simulink model "Framework"  (R2017b)
settings: Solver=ode1  StartTime=0.0  StopTime=Inf  FixedStep=0.001  RelTol=1e-3
PostLoadFcn:
  | , if any(exist('dsrtsu_mdlpostloadfcn', 'file') == [2, 3, 6]), try dsrtsu_mdlpostloadfcn('Execute', bdroot); catch fprintf('Error in PostLoadFcn (dsrtsu_mdlpostloadfcn) for model "%s":\n %s\n', bdroot, lasterr); end, end,
InitFcn:
  | Parameter_INIT
undefined symbols (not defined in the file or in its folder): drive, motor
libraries: rtican x46, simulink x8, neural x1
(part 10 of 10)

== system Framework/duty cycle RR/Transmit OK Detection ==
  note: This subsystem surveys if the sending of the TX message is successful and if it meets the
      | requirements concerning the regularity of the sending.
      |
      | If for 5 consecutive execution steps the message could not be successfully sent the 'TX Warn'
      | output is set to 1. Also, the message is expected to be sent every 50 ms approximatively. If this
      | condition is not met 5 times consecutively the 'TX Warn' output is set to 1.
  TX status : Inport
  TX delta time : Inport  Port=2
  Delta time limit : Constant  Value=0.055
  Delta time limit exceeded : RelationalOperator  RndMeth=Nearest  InputSameDT=on
  Mem{1..4} (4 alike) : Memory
  OR : Logic  Operator=OR
  Prev. msg. not sent : RelationalOperator  Operator=~=  RndMeth=Nearest  InputSameDT=on
  Prev. msg. sent value : Constant
  Warn : Logic  Inputs=5
  TX Warn : Outport
  wires:
  TX delta time/1 -> Delta time limit exceeded/1
  Delta time limit/1 -> Delta time limit exceeded/2
  Prev. msg. sent value/1 -> Prev. msg. not sent/2
  TX status/1 -> Prev. msg. not sent/1
  Prev. msg. not sent/1 -> OR/1
  Delta time limit exceeded/1 -> OR/2
  OR/1 -> Mem1/1, Warn/1
  Mem1/1 -> Mem2/1, Warn/2
  Mem2/1 -> Mem3/1, Warn/3
  Mem3/1 -> Mem4/1, Warn/4
  Mem4/1 -> Warn/5
  Warn/1 -> TX Warn/1

== system Framework/position FL/Transmit OK Detection ==
  note: This subsystem surveys if the sending of the TX message is successful and if it meets the
      | requirements concerning the regularity of the sending.
      |
      | If for 5 consecutive execution steps the message could not be successfully sent the 'TX Warn'
      | output is set to 1. Also, the message is expected to be sent every 50 ms approximatively. If this
      | condition is not met 5 times consecutively the 'TX Warn' output is set to 1.
  TX status : Inport
  TX delta time : Inport  Port=2
  Delta time limit : Constant  Value=0.055
  Delta time limit exceeded : RelationalOperator  RndMeth=Nearest  InputSameDT=on
  Mem{1..4} (4 alike) : Memory
  OR : Logic  Operator=OR
  Prev. msg. not sent : RelationalOperator  Operator=~=  RndMeth=Nearest  InputSameDT=on
  Prev. msg. sent value : Constant
  Warn : Logic  Inputs=5
  TX Warn : Outport
  wires:
  TX delta time/1 -> Delta time limit exceeded/1
  Delta time limit/1 -> Delta time limit exceeded/2
  Prev. msg. sent value/1 -> Prev. msg. not sent/2
  TX status/1 -> Prev. msg. not sent/1
  Prev. msg. not sent/1 -> OR/1
  Delta time limit exceeded/1 -> OR/2
  OR/1 -> Mem1/1, Warn/1
  Mem1/1 -> Mem2/1, Warn/2
  Mem2/1 -> Mem3/1, Warn/3
  Mem3/1 -> Mem4/1, Warn/4
  Mem4/1 -> Warn/5
  Warn/1 -> TX Warn/1

== system Framework/position FR/Transmit OK Detection ==
  note: This subsystem surveys if the sending of the TX message is successful and if it meets the
      | requirements concerning the regularity of the sending.
      |
      | If for 5 consecutive execution steps the message could not be successfully sent the 'TX Warn'
      | output is set to 1. Also, the message is expected to be sent every 50 ms approximatively. If this
      | condition is not met 5 times consecutively the 'TX Warn' output is set to 1.
  TX status : Inport
  TX delta time : Inport  Port=2
  Delta time limit : Constant  Value=0.055
  Delta time limit exceeded : RelationalOperator  RndMeth=Nearest  InputSameDT=on
  Mem{1..4} (4 alike) : Memory
  OR : Logic  Operator=OR
  Prev. msg. not sent : RelationalOperator  Operator=~=  RndMeth=Nearest  InputSameDT=on
  Prev. msg. sent value : Constant
  Warn : Logic  Inputs=5
  TX Warn : Outport
  wires:
  TX delta time/1 -> Delta time limit exceeded/1
  Delta time limit/1 -> Delta time limit exceeded/2
  Prev. msg. sent value/1 -> Prev. msg. not sent/2
  TX status/1 -> Prev. msg. not sent/1
  Prev. msg. not sent/1 -> OR/1
  Delta time limit exceeded/1 -> OR/2
  OR/1 -> Mem1/1, Warn/1
  Mem1/1 -> Mem2/1, Warn/2
  Mem2/1 -> Mem3/1, Warn/3
  Mem3/1 -> Mem4/1, Warn/4
  Mem4/1 -> Warn/5
  Warn/1 -> TX Warn/1

== system Framework/position RL/Transmit OK Detection ==
  note: This subsystem surveys if the sending of the TX message is successful and if it meets the
      | requirements concerning the regularity of the sending.
      |
      | If for 5 consecutive execution steps the message could not be successfully sent the 'TX Warn'
      | output is set to 1. Also, the message is expected to be sent every 50 ms approximatively. If this
      | condition is not met 5 times consecutively the 'TX Warn' output is set to 1.
  TX status : Inport
  TX delta time : Inport  Port=2
  Delta time limit : Constant  Value=0.055
  Delta time limit exceeded : RelationalOperator  RndMeth=Nearest  InputSameDT=on
  Mem{1..4} (4 alike) : Memory
  OR : Logic  Operator=OR
  Prev. msg. not sent : RelationalOperator  Operator=~=  RndMeth=Nearest  InputSameDT=on
  Prev. msg. sent value : Constant
  Warn : Logic  Inputs=5
  TX Warn : Outport
  wires:
  TX delta time/1 -> Delta time limit exceeded/1
  Delta time limit/1 -> Delta time limit exceeded/2
  Prev. msg. sent value/1 -> Prev. msg. not sent/2
  TX status/1 -> Prev. msg. not sent/1
  Prev. msg. not sent/1 -> OR/1
  Delta time limit exceeded/1 -> OR/2
  OR/1 -> Mem1/1, Warn/1
  Mem1/1 -> Mem2/1, Warn/2
  Mem2/1 -> Mem3/1, Warn/3
  Mem3/1 -> Mem4/1, Warn/4
  Mem4/1 -> Warn/5
  Warn/1 -> TX Warn/1

== system Framework/position RR/Transmit OK Detection ==
  note: This subsystem surveys if the sending of the TX message is successful and if it meets the
      | requirements concerning the regularity of the sending.
      |
      | If for 5 consecutive execution steps the message could not be successfully sent the 'TX Warn'
      | output is set to 1. Also, the message is expected to be sent every 50 ms approximatively. If this
      | condition is not met 5 times consecutively the 'TX Warn' output is set to 1.
  TX status : Inport
  TX delta time : Inport  Port=2
  Delta time limit : Constant  Value=0.055
  Delta time limit exceeded : RelationalOperator  RndMeth=Nearest  InputSameDT=on
  Mem{1..4} (4 alike) : Memory
  OR : Logic  Operator=OR
  Prev. msg. not sent : RelationalOperator  Operator=~=  RndMeth=Nearest  InputSameDT=on
  Prev. msg. sent value : Constant
  Warn : Logic  Inputs=5
  TX Warn : Outport
  wires:
  TX delta time/1 -> Delta time limit exceeded/1
  Delta time limit/1 -> Delta time limit exceeded/2
  Prev. msg. sent value/1 -> Prev. msg. not sent/2
  TX status/1 -> Prev. msg. not sent/1
  Prev. msg. not sent/1 -> OR/1
  Delta time limit exceeded/1 -> OR/2
  OR/1 -> Mem1/1, Warn/1
  Mem1/1 -> Mem2/1, Warn/2
  Mem2/1 -> Mem3/1, Warn/3
  Mem3/1 -> Mem4/1, Warn/4
  Mem4/1 -> Warn/5
  Warn/1 -> TX Warn/1

== system Framework/rpm FL/Transmit OK Detection1 ==
  note: This subsystem surveys if the sending of the TX message is successful and if it meets the
      | requirements concerning the regularity of the sending.
      |
      | If for 5 consecutive execution steps the message could not be successfully sent the 'TX Warn'
      | output is set to 1. Also, the message is expected to be sent every 50 ms approximatively. If this
      | condition is not met 5 times consecutively the 'TX Warn' output is set to 1.
  TX status : Inport
  TX delta time : Inport  Port=2
  Delta time limit : Constant  Value=0.055
  Delta time limit exceeded : RelationalOperator  RndMeth=Nearest  InputSameDT=on
  Mem{1..4} (4 alike) : Memory
  OR : Logic  Operator=OR
  Prev. msg. not sent : RelationalOperator  Operator=~=  RndMeth=Nearest  InputSameDT=on
  Prev. msg. sent value : Constant
  Warn : Logic  Inputs=5
  TX Warn : Outport
  wires:
  Warn/1 -> TX Warn/1
  Mem4/1 -> Warn/5
  Mem3/1 -> Warn/4, Mem4/1
  Mem2/1 -> Warn/3, Mem3/1
  Mem1/1 -> Warn/2, Mem2/1
  OR/1 -> Warn/1, Mem1/1
  Delta time limit exceeded/1 -> OR/2
  Prev. msg. not sent/1 -> OR/1
  TX status/1 -> Prev. msg. not sent/1
  Prev. msg. sent value/1 -> Prev. msg. not sent/2
  Delta time limit/1 -> Delta time limit exceeded/2
  TX delta time/1 -> Delta time limit exceeded/1

== system Framework/rpm FR/Transmit OK Detection1 ==
  note: This subsystem surveys if the sending of the TX message is successful and if it meets the
      | requirements concerning the regularity of the sending.
      |
      | If for 5 consecutive execution steps the message could not be successfully sent the 'TX Warn'
      | output is set to 1. Also, the message is expected to be sent every 50 ms approximatively. If this
      | condition is not met 5 times consecutively the 'TX Warn' output is set to 1.
  TX status : Inport
  TX delta time : Inport  Port=2
  Delta time limit : Constant  Value=0.055
  Delta time limit exceeded : RelationalOperator  RndMeth=Nearest  InputSameDT=on
  Mem{1..4} (4 alike) : Memory
  OR : Logic  Operator=OR
  Prev. msg. not sent : RelationalOperator  Operator=~=  RndMeth=Nearest  InputSameDT=on
  Prev. msg. sent value : Constant
  Warn : Logic  Inputs=5
  TX Warn : Outport
  wires:
  Warn/1 -> TX Warn/1
  Mem4/1 -> Warn/5
  Mem3/1 -> Warn/4, Mem4/1
  Mem2/1 -> Warn/3, Mem3/1
  Mem1/1 -> Warn/2, Mem2/1
  OR/1 -> Warn/1, Mem1/1
  Delta time limit exceeded/1 -> OR/2
  Prev. msg. not sent/1 -> OR/1
  TX status/1 -> Prev. msg. not sent/1
  Prev. msg. sent value/1 -> Prev. msg. not sent/2
  Delta time limit/1 -> Delta time limit exceeded/2
  TX delta time/1 -> Delta time limit exceeded/1

== system Framework/rpm RL/Transmit OK Detection1 ==
  note: This subsystem surveys if the sending of the TX message is successful and if it meets the
      | requirements concerning the regularity of the sending.
      |
      | If for 5 consecutive execution steps the message could not be successfully sent the 'TX Warn'
      | output is set to 1. Also, the message is expected to be sent every 50 ms approximatively. If this
      | condition is not met 5 times consecutively the 'TX Warn' output is set to 1.
  TX status : Inport
  TX delta time : Inport  Port=2
  Delta time limit : Constant  Value=0.055
  Delta time limit exceeded : RelationalOperator  RndMeth=Nearest  InputSameDT=on
  Mem{1..4} (4 alike) : Memory
  OR : Logic  Operator=OR
  Prev. msg. not sent : RelationalOperator  Operator=~=  RndMeth=Nearest  InputSameDT=on
  Prev. msg. sent value : Constant
  Warn : Logic  Inputs=5
  TX Warn : Outport
  wires:
  Warn/1 -> TX Warn/1
  Mem4/1 -> Warn/5
  Mem3/1 -> Warn/4, Mem4/1
  Mem2/1 -> Warn/3, Mem3/1
  Mem1/1 -> Warn/2, Mem2/1
  OR/1 -> Warn/1, Mem1/1
  Delta time limit exceeded/1 -> OR/2
  Prev. msg. not sent/1 -> OR/1
  TX status/1 -> Prev. msg. not sent/1
  Prev. msg. sent value/1 -> Prev. msg. not sent/2
  Delta time limit/1 -> Delta time limit exceeded/2
  TX delta time/1 -> Delta time limit exceeded/1

== system Framework/rpm RR/Transmit OK Detection1 ==
  note: This subsystem surveys if the sending of the TX message is successful and if it meets the
      | requirements concerning the regularity of the sending.
      |
      | If for 5 consecutive execution steps the message could not be successfully sent the 'TX Warn'
      | output is set to 1. Also, the message is expected to be sent every 50 ms approximatively. If this
      | condition is not met 5 times consecutively the 'TX Warn' output is set to 1.
  TX status : Inport
  TX delta time : Inport  Port=2
  Delta time limit : Constant  Value=0.055
  Delta time limit exceeded : RelationalOperator  RndMeth=Nearest  InputSameDT=on
  Mem{1..4} (4 alike) : Memory
  OR : Logic  Operator=OR
  Prev. msg. not sent : RelationalOperator  Operator=~=  RndMeth=Nearest  InputSameDT=on
  Prev. msg. sent value : Constant
  Warn : Logic  Inputs=5
  TX Warn : Outport
  wires:
  Warn/1 -> TX Warn/1
  Mem4/1 -> Warn/5
  Mem3/1 -> Warn/4, Mem4/1
  Mem2/1 -> Warn/3, Mem3/1
  Mem1/1 -> Warn/2, Mem2/1
  OR/1 -> Warn/1, Mem1/1
  Delta time limit exceeded/1 -> OR/2
  Prev. msg. not sent/1 -> OR/1
  TX status/1 -> Prev. msg. not sent/1
  Prev. msg. sent value/1 -> Prev. msg. not sent/2
  Delta time limit/1 -> Delta time limit exceeded/2
  TX delta time/1 -> Delta time limit exceeded/1

== system Framework/RTI Data/RTI Data Store/RTI Data Store ==
  RTI Data Store : Subsystem  mask(RTI_DATA_STORE){}
      mask help:
      | RTI Data Store Block. This block is used by RTI to store internal model dependent data. Deleting this block will result in data loss.
      |
      | NEVER DELETE, COPY, OR MODIFY THIS BLOCK!
      mask Help:
      | RTI Data Store Block. This block is used by RTI to store internal model dependent data. Deleting this block will result in data loss.
      | 
      | NEVER DELETE, COPY, OR MODIFY THIS BLOCK!
      mask Display: text(0.5, 0.5, ' ', 'HorizontalAlignment', 'center');

== system Framework/RTI Data/RTI Data Store/RTI Data Store/RTI Data Store ==
  RTI Data Store : Subsystem  mask(RTI_DATA_STORE){}
      mask help:
      | RTI Data Store Block. This block is used by RTI to store internal model dependent data. Deleting this block will result in data loss.
      |
      | NEVER DELETE, COPY, OR MODIFY THIS BLOCK!
      mask Help:
      | RTI Data Store Block. This block is used by RTI to store internal model dependent data. Deleting this block will result in data loss.
      | 
      | NEVER DELETE, COPY, OR MODIFY THIS BLOCK!
      mask Display: text(0.5, 0.5, ' ', 'HorizontalAlignment', 'center');

== system Framework/RTI Data/RTI Data Store/RTI Data Store/RTI Data Store/RTI Data Store ==
